simulink model "test_transformers"  (R2025b)
settings: Solver=VariableStepAuto  StartTime=0.0  StopTime=5/60  RelTol=1e-3
libraries: fl_lib x31, ee_lib_for_power_systems x27, nesl_utility x7, ee_lib x4, custom_lib x3
settings Model: SimulationMode=accelerator  Creator=gdudgeon  LastModifiedBy=gdudgeon
settings RTWCC: GPUComputeCapability=3.5

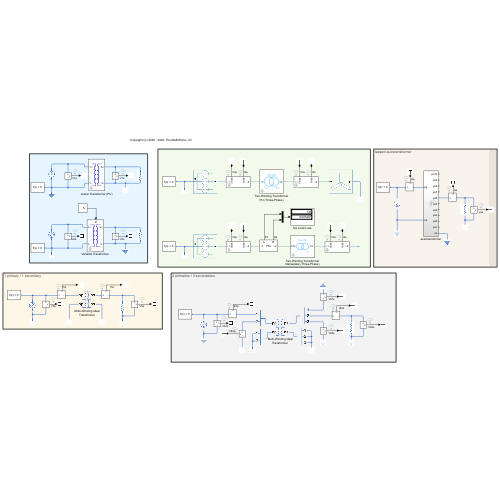
[thumbnail: Simulink's stored preview of the top-level diagram]
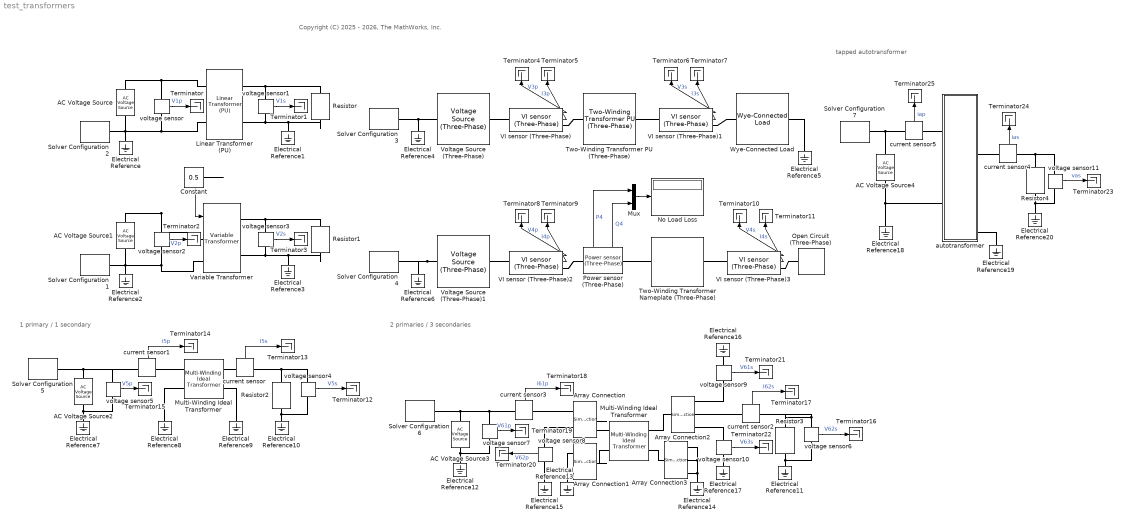
== system test_transformers ==
  note: tapped autotransformer
  note: 1 primary / 1 secondary
  note: Copyright (C) 2025 - 2026, The MathWorks, Inc.
  note: 2 primaries / 3 secondaries
  AC Voltage Source : fl_lib/Electrical/Electrical Sources/AC Voltage Source  amp=100000*sqrt(3/2) V  shift=0 deg  frequency=60 Hz
  AC Voltage Source1 : fl_lib/Electrical/Electrical Sources/AC Voltage Source  amp=100000*sqrt(3/2) V  shift=0 deg  frequency=60 Hz
  AC Voltage Source2 : fl_lib/Electrical/Electrical Sources/AC Voltage Source  amp=100 V  shift=0 deg  frequency=60 Hz
  AC Voltage Source3 : fl_lib/Electrical/Electrical Sources/AC Voltage Source  amp=100 V  shift=0 deg  frequency=60 Hz
  AC Voltage Source4 : fl_lib/Electrical/Electrical Sources/AC Voltage Source  amp=100 V  shift=0 deg  frequency=60 Hz
  Array Connection : SimscapeArrayConnection
  Array Connection1 : SimscapeArrayConnection
  Array Connection2 : SimscapeArrayConnection  NumScalarElements=3
  Array Connection3 : SimscapeArrayConnection  NumScalarElements=3
  Constant : Constant  Value=0.5
  Electrical Reference{,1..20} (21 alike) : fl_lib/Electrical/Electrical Elements/Electrical Reference
  Linear Transformer (PU) : ee_lib_for_power_systems/Network Components/Linear Transformer (PU)  Pnom_Fnom=[100e6 60]  V1_V2=[100000 50000]  R_X=[0.01 0.08]  Rm_Xm=[500 500]  run_time=off
      settings: SourceProductName=Support Library for Power Systems
  Multi-Winding Ideal Transformer : custom_lib/Multi-Winding Ideal Transformer  npw=1  nsw=1  nVp=100 V  nVs=200 V
      settings: InternalSimscapePortConfiguration="{\"Bottom\":[],\"Left\":[{\"id\":\"pp\",\"label\":\"pp\",\"type\":\"foundation.electrical.electrical\"},{\"id\":\"np\",\"label\":\"np\",\"type\":\"foundation.electrical.electrical\"}],\"Right\":[{\"id\":\"ps\",\"label\":\"ps\",\"type\":\"foundation.electrical.electrical\"},{\"id\":\"ns\",\"label\":\"ns\",\"type\":\"foundation.electrical.electrical\"}],\"Top\":[]}"
  "Multi-Winding Ideal Transformer " : custom_lib/Multi-Winding Ideal Transformer  npw=2  nsw=3  nVp=[100 50] V  nVs=[200 300 400] V
      settings: InternalSimscapePortConfiguration="{\"Bottom\":[],\"Left\":[{\"id\":\"pp\",\"label\":\"pp\",\"type\":\"foundation.electrical.electrical\"},{\"id\":\"np\",\"label\":\"np\",\"type\":\"foundation.electrical.electrical\"}],\"Right\":[{\"id\":\"ps\",\"label\":\"ps\",\"type\":\"foundation.electrical.electrical\"},{\"id\":\"ns\",\"label\":\"ns\",\"type\":\"foundation.electrical.electrical\"}],\"Top\":[]}"
  Mux : Mux  Inputs=2
  No Load Loss : Display
  Open Circuit (Three-Phase) : ee_lib/Connectors & References/Open Circuit (Three-Phase)
      settings: InternalSimscapePortConfiguration="{\"Bottom\":[],\"Left\":[{\"id\":\"N\",\"label\":\"~\",\"type\":\"foundation.electrical.three_phase\"}],\"Right\":[],\"Top\":[]}"
  Power sensor (Three-Phase) : ee_lib_for_power_systems/Sense and Measure/Power sensor (Three-Phase)  SystemSampleTime=-1  VariantActivationTime=update diagram  EmptyChoice=off  PassThrough=off  PassThroughVariantControl=(default)  EmptyChoiceVariantControl=(default)  AllowFlexibleInterface=on  Latency=0  AutoFrameSizeCalculation=off
      settings: SourceProductName=Support Library for Power Systems  PortSchema="{\"entries\":[{\"content\":{\"sides\":[{\"content\":{\"connectorIds\":[\"LConn1\"]},\"type\":\"ConnectorPlacement.EquallySpacedRectSide\",\"uuid\":\"d536c57f-d596-4c30-b2f2-ca7a7128ca09\"},{\"content\":{\"connectorIds\":[\"RConn1\"],\"side\":\"RIGHT\"},\"type\":\"ConnectorPlacement.EquallySpacedRectSide\",\"uuid\":\"3e38bcb4-aad6-4c8e-8ba0-f34fad0d941d\"},{\"content\":{\"connectorIds\":[\"Out1\",\"Out2\"],\"side\":\"TOP\"},\"type\":\"ConnectorPlacement.EquallySpacedRectSide\",\"uuid\":\"dbbb5dbf-676f-46fa-997f-a90b77759865\"}]},\"type\":\"ConnectorPlacement.EquallySpacedConnector\",\"uuid\":\"d250c4d3-27c8-4176-913c-392fad876444\"}],\"packageUris\":[\"http://schema.mathworks.com/mf0/Connector/R2020b\"],\"version\":\"1.0\"}"
  Resistor : fl_lib/Electrical/Electrical Elements/Resistor  R=1e5 Ohm  i_specify=off  i_priority=None  i=0 A  i_nominal_specify=off  i_nominal_value=1  i_nominal_unit=A  v_specify=off  v_priority=None  v=0 V  v_nominal_specify=off  v_nominal_value=1  v_nominal_unit=V
  Resistor1 : fl_lib/Electrical/Electrical Elements/Resistor  R=1e5 Ohm  i_specify=off  i_priority=None  i=0 A  i_nominal_specify=off  i_nominal_value=1  i_nominal_unit=A  v_specify=off  v_priority=None  v=0 V  v_nominal_specify=off  v_nominal_value=1  v_nominal_unit=V
  Resistor2 : fl_lib/Electrical/Electrical Elements/Resistor  R=1 Ohm  i_specify=off  i_priority=None  i=0 A  i_nominal_specify=off  i_nominal_value=1  i_nominal_unit=A  v_specify=off  v_priority=None  v=0 V  v_nominal_specify=off  v_nominal_value=1  v_nominal_unit=V
  Resistor3 : fl_lib/Electrical/Electrical Elements/Resistor  R=1 Ohm  i_specify=off  i_priority=None  i=0 A  i_nominal_specify=off  i_nominal_value=1  i_nominal_unit=A  v_specify=off  v_priority=None  v=0 V  v_nominal_specify=off  v_nominal_value=1  v_nominal_unit=V
  Resistor4 : fl_lib/Electrical/Electrical Elements/Resistor  R=1 Ohm  i_specify=off  i_priority=None  i=0 A  i_nominal_specify=off  i_nominal_value=1  i_nominal_unit=A  v_specify=off  v_priority=None  v=0 V  v_nominal_specify=off  v_nominal_value=1  v_nominal_unit=V
  Solver Configuration {1..7} (7 alike) : nesl_utility/Solver Configuration  PhysicalDomain=network_engine_domain  SubClassName=solver  LeftPortType=input  RightPortType=generic  Tones=[]  Harmonics=[]  SimulateNoise=off  Profile=off  UseLocalSampling=off  EnableSwitchedLinearOptims=on  FrequencyDomain=off  UseCCode=off  RelTol=0.001  AbsTol=0.001  MinStep=1e-09  ToWorkspace=off  RevertToSquareIcSolve=off  NumHomotopyIterations=100  PhasorMode=off  PhasorModeNumHarmonics=1  ConsistencySolver=NEWTON_XTOL_AFTER_FTOL  IndexReductionMethod=None  DoDC=off  ResidualTolerance=1e-09  ConsistencyTolSource=GLOBAL  ConsistencyAbsTol=0.001  ConsistencyRelTol=0.001  ConsistencyTolFactor=0.001  UseLocalSolver=on  LocalSolverChoice=NE_PARTITIONING_ADVANCER  ResolveIndetEquations=off  FunctionEvalNumThread=1  LocalSolverSampleTime=50e-6  DoFixedCost=off  MaxNonlinIter=2  MaxModeIter=2  ComputeImpulses=off  ImpulseIterations=2  LinearAlgebra=Sparse  LinearAlgebraNumThread=0  EquationFormulation=NE_TIME_EF  DelaysMemoryBudget=1024  AutomaticFiltering=off  FilteringTimeConstant=0.001  PartitionStorageMethod=AS_NEEDED  PartitionMemoryBudget=1024  PartitionMethod=ROBUST  MultibodyUseLocalSolver=off  MultibodyLocalSolverChoice=ODE1  MultibodyLocalSolverSampleTime=0.001
  Terminator{,1..25} (26 alike) : Terminator
  Two-Winding Transformer Nameplate (Three-Phase) : ee_lib_for_power_systems/Network Components/Two-Winding Transformer Nameplate (Three-Phase)  conn1=Y  conn2=Y  core=threelimb  Prated=100  Frated=60  HV_LV=[11000 415]  HVA_LVA=[5.25 139.1]  Zperc=3.88  load_loss=1750  no_load_loss=145  run_time=off
      settings: SourceProductName=Support Library for Power Systems
  Two-Winding Transformer PU (Three-Phase) : ee_lib_for_power_systems/Network Components/Two-Winding Transformer PU (Three-Phase)  conn1=Yg  conn2=delta1  core=threelimb  Pnom_Fnom=[250e6 60]  V1_V2=[500000 250000]  R_X=[0.01 0.05]  Rm_Xm=[500 500]  run_time=on
      settings: SourceProductName=Support Library for Power Systems
  VI sensor (Three-Phase){,1..3} (4 alike) : ee_lib_for_power_systems/Sense and Measure/VI sensor (Three-Phase)  volt_meas=Line-to-Line (Line Voltage)  meas_units=SI  Vnom=24e3  Pnom=100e6
      settings: SourceProductName=Support Library for Power Systems
  Variable Transformer : ee_lib_for_power_systems/Network Components/Variable Transformer
      settings: SourceProductName=Support Library for Power Systems
  Voltage Source (Three-Phase) : ee_lib/Sources/Voltage Source (Three-Phase)  vline_rms=100e3 V  shift=0 deg  freq=60 Hz  impedance_option=0  SShortCircuit=1e6 A*V  XR=15  R=0.01 Ohm  L=3.97e-4 H  harmonic_option=0  harmonic_orders=[5, 7, 11, 13]  harmonic_ratios=[.1, .1, .1, .1]  G_parasitic=0 1/Ohm  I_specify=off  I_priority=None  I=[0, 0, 0] A  I_nominal_specify=off  I_nominal_value=1  I_nominal_unit=A
  Voltage Source (Three-Phase)1 : ee_lib/Sources/Voltage Source (Three-Phase)  vline_rms=11e3 V  shift=0 deg  freq=60 Hz  impedance_option=0  SShortCircuit=1e6 A*V  XR=15  R=0.01 Ohm  L=3.97e-4 H  harmonic_option=0  harmonic_orders=[5, 7, 11, 13]  harmonic_ratios=[.1, .1, .1, .1]  G_parasitic=0 1/Ohm  I_specify=off  I_priority=None  I=[0, 0, 0] A  I_nominal_specify=off  I_nominal_value=1  I_nominal_unit=A
  Wye-Connected Load : ee_lib/Passive/RLC Assemblies/Wye-Connected Load  port_option=ee.enum.threePhasePort.composite  parameterization=ee.enum.rlc.parameterization.ratedpower  component_structure=ee.enum.rlc.structure.R  component_structure_PQ=ee.enum.rlc.structure.R  R=1 Ohm  L=1e-3 H  C=1e-6 F  VRated=100e3 V  FRated=60 Hz  P=1e3 W  Qpos=1e2 A*V  Qneg=-1e2 A*V  R_parasitic=0 Ohm  G_parasitic=0 1/Ohm  R_parasitic_PQ=0 Ohm  G_parasitic_PQ=0 1/Ohm  Vmag0=24e3 V  Vang0=0 deg  Freq0=60 Hz  IL_specify=off  IL_priority=High  IL=[0, 0, 0] A  IL_nominal_specify=off  IL_nominal_value=1  IL_nominal_unit=A  VC_specify=off  VC_priority=High  VC=[0, 0, 0] V  VC_nominal_specify=off  VC_nominal_value=1  VC_nominal_unit=V
  autotransformer : Subsystem
  current sensor{,1..5} (6 alike) : ee_lib_for_power_systems/Sense and Measure/current sensor  SystemSampleTime=-1  VariantActivationTime=update diagram  EmptyChoice=off  PassThrough=off  PassThroughVariantControl=(default)  EmptyChoiceVariantControl=(default)  AllowFlexibleInterface=on  Latency=0  AutoFrameSizeCalculation=off
      settings: SourceProductName=Support Library for Power Systems  PortSchema="{\"entries\":[{\"content\":{\"sides\":[{\"content\":{\"connectorIds\":[\"LConn1\"]},\"type\":\"ConnectorPlacement.EquallySpacedRectSide\",\"uuid\":\"799648ba-196f-427a-9565-f64fffdae700\"},{\"content\":{\"connectorIds\":[\"RConn1\"],\"side\":\"RIGHT\"},\"type\":\"ConnectorPlacement.EquallySpacedRectSide\",\"uuid\":\"662de5d5-c2ef-406c-9235-94a35f9d89fb\"},{\"content\":{\"connectorIds\":[\"Out1\"],\"side\":\"TOP\"},\"type\":\"ConnectorPlacement.EquallySpacedRectSide\",\"uuid\":\"67dc8fec-98bd-426f-bbe6-5723f2587b12\"}]},\"type\":\"ConnectorPlacement.EquallySpacedConnector\",\"uuid\":\"3e33dbb3-529a-4788-9727-18d62c402281\"}],\"packageUris\":[\"http://schema.mathworks.com/mf0/Connector/R2020b\"],\"version\":\"1.0\"}"
  voltage sensor{,1..11} (12 alike) : ee_lib_for_power_systems/Sense and Measure/voltage sensor  SystemSampleTime=-1  VariantActivationTime=update diagram  EmptyChoice=off  PassThrough=off  PassThroughVariantControl=(default)  EmptyChoiceVariantControl=(default)  AllowFlexibleInterface=on  Latency=0  AutoFrameSizeCalculation=off
      settings: SourceProductName=Support Library for Power Systems  PortSchema="{\"entries\":[{\"content\":{\"sides\":[{\"content\":{},\"type\":\"ConnectorPlacement.EquallySpacedRectSide\",\"uuid\":\"799648ba-196f-427a-9565-f64fffdae700\"},{\"content\":{\"connectorIds\":[\"Out1\"],\"side\":\"RIGHT\"},\"type\":\"ConnectorPlacement.EquallySpacedRectSide\",\"uuid\":\"662de5d5-c2ef-406c-9235-94a35f9d89fb\"},{\"content\":{\"connectorIds\":[\"LConn1\"],\"side\":\"TOP\"},\"type\":\"ConnectorPlacement.EquallySpacedRectSide\",\"uuid\":\"67dc8fec-98bd-426f-bbe6-5723f2587b12\"},{\"content\":{\"connectorIds\":[\"RConn1\"],\"side\":\"BOTTOM\"},\"type\":\"ConnectorPlacement.EquallySpacedRectSide\",\"uuid\":\"7e3d7354-1ab6-44d8-9b44-c988118d052c\"}]},\"type\":\"ConnectorPlacement.EquallySpacedConnector\",\"uuid\":\"3e33dbb3-529a-4788-9727-18d62c402281\"}],\"packageUris\":[\"http://schema.mathworks.com/mf0/Connector/R2020b\"],\"version\":\"1.0\"}"
  wires:
  voltage sensor/1 -> Terminator/1  "V1p"
  voltage sensor1/1 -> Terminator1/1  "V1s"
  voltage sensor3/1 -> Terminator3/1  "V2s"
  voltage sensor2/1 -> Terminator2/1  "V2p"
  Constant/1 -> Variable Transformer/1
  VI sensor (Three-Phase)/1 -> Terminator4/1  "V3p"
  VI sensor (Three-Phase)/2 -> Terminator5/1  "I3p"
  VI sensor (Three-Phase)1/1 -> Terminator6/1  "V3s"
  VI sensor (Three-Phase)1/2 -> Terminator7/1  "I3s"
  VI sensor (Three-Phase)3/2 -> Terminator11/1  "I4s"
  VI sensor (Three-Phase)3/1 -> Terminator10/1  "V4s"
  VI sensor (Three-Phase)2/2 -> Terminator9/1  "I4p"
  VI sensor (Three-Phase)2/1 -> Terminator8/1  "V4p"
  Power sensor (Three-Phase)/1 -> Mux/1  "P4"
  Power sensor (Three-Phase)/2 -> Mux/2  "Q4"
  Mux/1 -> No Load Loss/1
  voltage sensor4/1 -> Terminator12/1  "V5s"
  current sensor/1 -> Terminator13/1  "I5s"
  current sensor1/1 -> Terminator14/1  "i5p"
  voltage sensor5/1 -> Terminator15/1  "V5p"
  voltage sensor7/1 -> Terminator19/1  "V61p"
  current sensor3/1 -> Terminator18/1  "i61p"
  current sensor2/1 -> Terminator17/1  "I62s"
  voltage sensor6/1 -> Terminator16/1  "V62s"
  voltage sensor8/1 -> Terminator20/1  "V62p"
  voltage sensor9/1 -> Terminator21/1  "V61s"
  voltage sensor10/1 -> Terminator22/1  "V63s"
  voltage sensor11/1 -> Terminator23/1  "vas"
  current sensor4/1 -> Terminator24/1  "ias"
  current sensor5/1 -> Terminator25/1  "iap"
  connections:
  AC Voltage Source/LConn1 -- Linear Transformer (PU)/LConn1 -- voltage sensor/LConn1
  AC Voltage Source/RConn1 -- Linear Transformer (PU)/LConn2 -- voltage sensor/RConn1 -- Solver Configuration 2/RConn1 -- Electrical Reference/LConn1
  Linear Transformer (PU)/RConn1 -- voltage sensor1/LConn1 -- Resistor/LConn1
  Resistor/RConn1 -- Electrical Reference1/LConn1 -- Linear Transformer (PU)/RConn2 -- voltage sensor1/RConn1
  voltage sensor2/LConn1 -- AC Voltage Source1/LConn1 -- Variable Transformer/LConn1
  AC Voltage Source1/RConn1 -- Electrical Reference2/LConn1 -- Solver Configuration 1/RConn1 -- voltage sensor2/RConn1 -- Variable Transformer/LConn2
  voltage sensor3/LConn1 -- Variable Transformer/RConn1 -- Resistor1/LConn1
  Electrical Reference3/LConn1 -- Resistor1/RConn1 -- voltage sensor3/RConn1 -- Variable Transformer/RConn2
  Electrical Reference4/LConn1 -- Voltage Source (Three-Phase)/LConn1 -- Solver Configuration 3/RConn1
  VI sensor (Three-Phase)/LConn1 -- Voltage Source (Three-Phase)/RConn1
  Two-Winding Transformer PU (Three-Phase)/LConn1 -- VI sensor (Three-Phase)/RConn1
  VI sensor (Three-Phase)1/LConn1 -- Two-Winding Transformer PU (Three-Phase)/RConn1
  Wye-Connected Load/LConn1 -- VI sensor (Three-Phase)1/RConn1
  Electrical Reference5/LConn1 -- Wye-Connected Load/RConn1
  Voltage Source (Three-Phase)1/LConn1 -- Electrical Reference6/LConn1 -- Solver Configuration 4/RConn1
  Open Circuit (Three-Phase)/LConn1 -- VI sensor (Three-Phase)3/RConn1
  Two-Winding Transformer Nameplate (Three-Phase)/RConn1 -- VI sensor (Three-Phase)3/LConn1
  VI sensor (Three-Phase)2/LConn1 -- Voltage Source (Three-Phase)1/RConn1
  Power sensor (Three-Phase)/LConn1 -- VI sensor (Three-Phase)2/RConn1
  Power sensor (Three-Phase)/RConn1 -- Two-Winding Transformer Nameplate (Three-Phase)/LConn1
  AC Voltage Source2/LConn1 -- current sensor1/LConn1 -- voltage sensor5/LConn1 -- Solver Configuration 5/RConn1
  Electrical Reference8/LConn1 -- Multi-Winding Ideal Transformer/LConn2
  Electrical Reference7/LConn1 -- voltage sensor5/RConn1 -- AC Voltage Source2/RConn1
  Electrical Reference9/LConn1 -- Multi-Winding Ideal Transformer/RConn2
  Resistor2/LConn1 -- voltage sensor4/LConn1 -- current sensor/RConn1
  Electrical Reference10/LConn1 -- voltage sensor4/RConn1 -- Resistor2/RConn1
  current sensor/LConn1 -- Multi-Winding Ideal Transformer/RConn1
  current sensor1/RConn1 -- Multi-Winding Ideal Transformer/LConn1
  current sensor3/LConn1 -- voltage sensor7/LConn1 -- AC Voltage Source3/LConn1 -- Solver Configuration 6/RConn1
  voltage sensor7/RConn1 -- Electrical Reference12/LConn1 -- AC Voltage Source3/RConn1
  voltage sensor6/LConn1 -- Resistor3/LConn1 -- current sensor2/RConn1
  voltage sensor6/RConn1 -- Electrical Reference11/LConn1 -- Resistor3/RConn1
  Array Connection/RConn1 -- "Multi-Winding Ideal Transformer "/LConn1
  Array Connection1/RConn1 -- "Multi-Winding Ideal Transformer "/LConn2
  "Multi-Winding Ideal Transformer "/RConn1 -- Array Connection2/RConn1
  "Multi-Winding Ideal Transformer "/RConn2 -- Array Connection3/RConn1
  Electrical Reference13/LConn1 -- Array Connection1/LConn2 -- Array Connection1/LConn1
  Electrical Reference14/LConn1 -- Array Connection3/LConn1 -- Array Connection3/LConn2 -- Array Connection3/LConn3
  current sensor2/LConn1 -- Array Connection2/LConn2
  current sensor3/RConn1 -- Array Connection/LConn1
  voltage sensor8/LConn1 -- Array Connection/LConn2
  Electrical Reference15/LConn1 -- voltage sensor8/RConn1
  Array Connection2/LConn1 -- voltage sensor9/LConn1
  Electrical Reference16/LConn1 -- voltage sensor9/RConn1
  voltage sensor10/LConn1 -- Array Connection2/LConn3
  Electrical Reference17/LConn1 -- voltage sensor10/RConn1
  AC Voltage Source4/LConn1 -- current sensor5/LConn1 -- Solver Configuration 7/RConn1
  AC Voltage Source4/RConn1 -- Electrical Reference18/LConn1 -- autotransformer/LConn2
  Electrical Reference19/LConn1 -- autotransformer/RConn11
  Electrical Reference20/LConn1 -- voltage sensor11/RConn1 -- Resistor4/RConn1
  Resistor4/LConn1 -- current sensor4/RConn1 -- voltage sensor11/LConn1
  current sensor5/RConn1 -- autotransformer/LConn1
  current sensor4/LConn1 -- autotransformer/RConn5

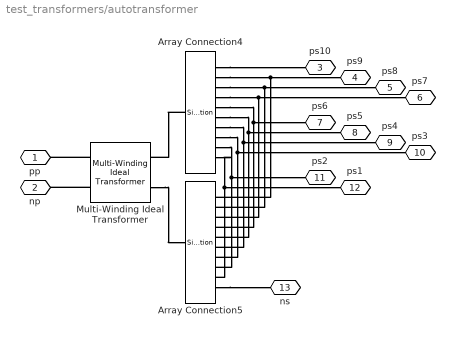
== system test_transformers/autotransformer ==
  Array Connection4 : SimscapeArrayConnection  NumScalarElements=10
  Array Connection5 : SimscapeArrayConnection  NumScalarElements=10
  Multi-Winding Ideal Transformer : custom_lib/Multi-Winding Ideal Transformer  npw=1  nsw=10  nVp=10 V  nVs=ones(1,10) V
      settings: InternalSimscapePortConfiguration="{\"Bottom\":[],\"Left\":[{\"id\":\"pp\",\"label\":\"pp\",\"type\":\"foundation.electrical.electrical\"},{\"id\":\"np\",\"label\":\"np\",\"type\":\"foundation.electrical.electrical\"}],\"Right\":[{\"id\":\"ps\",\"label\":\"ps\",\"type\":\"foundation.electrical.electrical\"},{\"id\":\"ns\",\"label\":\"ns\",\"type\":\"foundation.electrical.electrical\"}],\"Top\":[]}"
  pp : PMIOPort  Side=Left
  np : PMIOPort  Port=2  Side=Left
  ps10 : PMIOPort  Port=3  Side=Right
  ps9 : PMIOPort  Port=4  Side=Right
  ps8 : PMIOPort  Port=5  Side=Right
  ps7 : PMIOPort  Port=6  Side=Right
  ps6 : PMIOPort  Port=7  Side=Right
  ps5 : PMIOPort  Port=8  Side=Right
  ps4 : PMIOPort  Port=9  Side=Right
  ps3 : PMIOPort  Port=10  Side=Right
  ps2 : PMIOPort  Port=11  Side=Right
  ps1 : PMIOPort  Port=12  Side=Right
  ns : PMIOPort  Port=13  Side=Right
  connections:
  Multi-Winding Ideal Transformer/LConn1 -- pp/RConn1
  Multi-Winding Ideal Transformer/RConn2 -- Array Connection5/RConn1
  Array Connection4/LConn2 -- ps9/RConn1 -- Array Connection5/LConn1
  Array Connection4/LConn4 -- Array Connection5/LConn3 -- ps7/RConn1
  Array Connection4/LConn8 -- Array Connection5/LConn7 -- ps3/RConn1
  Array Connection4/LConn10 -- Array Connection5/LConn9 -- ps1/RConn1
  Array Connection4/LConn6 -- Array Connection5/LConn5 -- ps5/RConn1
  Array Connection4/LConn5 -- ps6/RConn1 -- Array Connection5/LConn4
  Array Connection4/RConn1 -- Multi-Winding Ideal Transformer/RConn1
  Array Connection4/LConn9 -- Array Connection5/LConn8 -- ps2/RConn1
  Array Connection4/LConn7 -- Array Connection5/LConn6 -- ps4/RConn1
  Array Connection4/LConn3 -- Array Connection5/LConn2 -- ps8/RConn1
  Array Connection5/LConn10 -- ns/RConn1
  Multi-Winding Ideal Transformer/LConn2 -- np/RConn1
  Array Connection4/LConn1 -- ps10/RConn1
